simulink model "modulacaoqpsk"  (R2015a)
settings: Solver=FixedStepDiscrete  StartTime=0.0  StopTime=10.0  RelTol=1e-3
libraries: dspsrcs4 x2, simulink x1, commdigbbndpm3 x1
settings Model: Creator=jessica.c13  LastModifiedBy=jessica.c13
settings OptimizationCC: BlockReduction=off  ConditionallyExecuteInputs=off  InlineParams=on
settings DebuggingCC: AlgebraicLoopMsg=error
settings HardwareCC: ProdHWDeviceType=ASIC/FPGA->ASIC/FPGA  ProdEqTarget=off

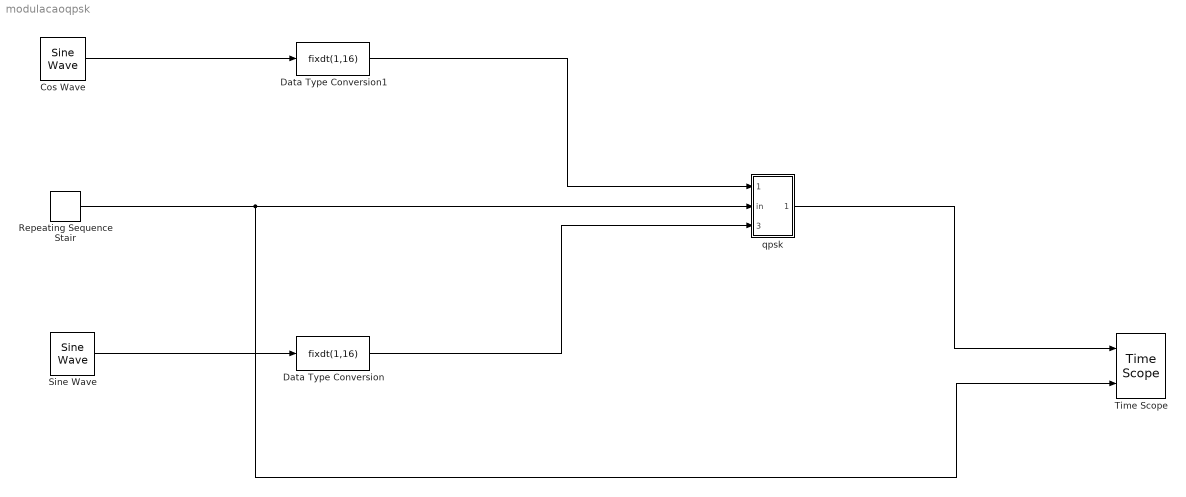
== system modulacaoqpsk ==
  Cos Wave : dspsrcs4/Sine Wave  Amplitude=1  Frequency=4  Phase=pi/2  SampleMode=Discrete  OutComplex=Real  CompMethod=Trigonometric fcn  TableSize=Speed  SampleTime=1/100  SamplesPerFrame=1  ResetState=Restart at time zero  dataType=double  wordLen=16  udDataType=sfix(16)  fracBitsMode=Best precision  numFracBits=15  OutDataTypeStr=double  LastOutDataTypeStr=double
  Data Type Conversion : DataTypeConversion  OutMin=-1  OutMax=1  OutDataTypeStr=fixdt(1,16)
  Data Type Conversion1 : DataTypeConversion  OutMin=-1  OutMax=1  OutDataTypeStr=fixdt(1,16)
  Repeating Sequence Stair : simulink/Sources/Repeating Sequence Stair  OutValues=[0 0 0 0 0 0 0 0 0 0 0 0 0 0 0 0 0 0 0 0 0 0 0 0 0 0 0 0 0 0 0 0 0 0 0 0 0 0 0 0 0 0 0 0 0 0 0 0 0 0 1 1 1 1 1 1 1 1 1 1 1 1 1 1 1 1 1 1 1 1 1 1 1 1 1 1 1 1 1 1 1 1 1 1 1 1 1 1 1 1 1 1 1 1 1 1 1 1 1 1 2 2 2 2 2 2 2 2 2 2 2 2 2 2 2 2 2 2 2 2 2 2 2 2 2 2 2 2 2 2 2 2 2 2 2 2 2 2 2 2 2 2 2 2 2 2 2 2 2 2 3 3 3 3 3 3 3 3 3 3 3 3 3 3 3 3 3 3 3 3 3 3 3 3 3 3 3 3 3 3 3 3 3 3 3 3 3 3 3 3 3 3 3 3 3 3 3 3 3 3].'  tsamp=1/100  OutMin=0  OutMax=3  OutDataTypeStr=int8  OutputDataTypeScalingMode=int8  OutDataType=fixdt(0,8)  ConRadixGroup=Best Precision: Vector-wise  OutScaling=2^-12
  Sine Wave : dspsrcs4/Sine Wave  Amplitude=1  Frequency=4  Phase=0  SampleMode=Discrete  OutComplex=Real  CompMethod=Trigonometric fcn  TableSize=Speed  SampleTime=1/100  SamplesPerFrame=1  ResetState=Restart at time zero  dataType=double  wordLen=16  udDataType=sfix(16)  fracBitsMode=Best precision  numFracBits=15  OutDataTypeStr=double  LastOutDataTypeStr=double
  Time Scope : TimeScope  DefaultConfigurationName=spbscopes.TimeScopeBlockCfg  NumInputPorts=2
  qpsk : Subsystem
  wires:
  Sine Wave/1 -> Data Type Conversion/1
  Cos Wave/1 -> Data Type Conversion1/1
  Repeating Sequence Stair/1 -> Time Scope/2, qpsk/2(in)
  Data Type Conversion1/1 -> qpsk/1(cos)
  Data Type Conversion/1 -> qpsk/3(sen)
  qpsk/1(out) -> Time Scope/1

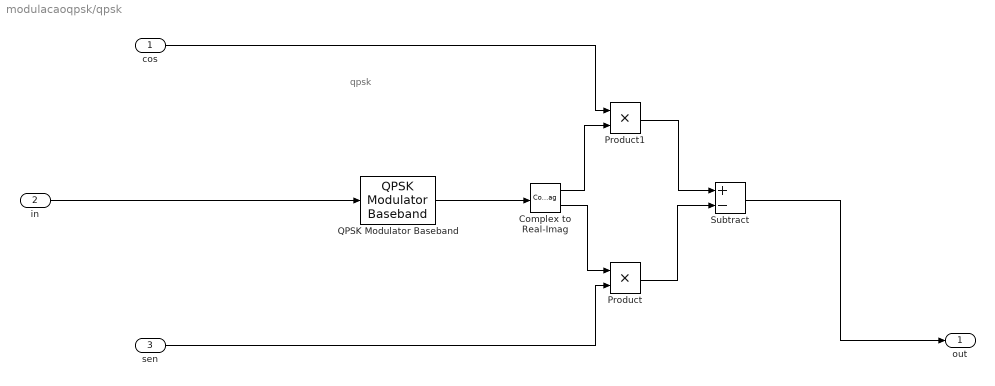
== system modulacaoqpsk/qpsk ==
  note: qpsk
  cos : Inport
  in : Inport  Port=2
  sen : Inport  Port=3
  Complex to Real-Imag : ComplexToRealImag
  Product : Product
  Product1 : Product
  QPSK Modulator Baseband : commdigbbndpm3/QPSK Modulator Baseband  InType=Integer  Enc=Gray  Ph=0  outDtype=Fixed-point  outWordLen=8  outUDDataType=sfix(16)  outFracLenMode=Best precision  outFracLen=15
  Subtract : Sum  Inputs=+-
  out : Outport
  wires:
  Complex to Real-Imag/1 -> Product1/2
  QPSK Modulator Baseband/1 -> Complex to Real-Imag/1
  sen/1 -> Product/2
  Subtract/1 -> out/1
  Product1/1 -> Subtract/1
  cos/1 -> Product1/1
  Complex to Real-Imag/2 -> Product/1
  Product/1 -> Subtract/2
  in/1 -> QPSK Modulator Baseband/1
